simulink model "ex_codegen_dsp"  (R2013a)
settings: Solver=FixedStepDiscrete  SolverMode=SingleTasking  StartTime=0.0  StopTime=60  RelTol=1e-3
undefined symbols (not defined in the file or in its folder): fdesignblkfcn, gcbh, get
libraries: dspsrcs4 x2, dspadpt3 x1, dspsnks4 x1
CloseFcn:
  | clear filter_wts;
  | clear tout;
settings Model: Creator=The MathWorks Inc.  LastModifiedBy=mainster
settings DataIOCC: SignalLoggingSaveFormat=ModelDataLogs
settings OptimizationCC: ExpressionDepthLimit=2147483647
settings DebuggingCC: FcnCallInpInsideContextMsg=UseLocalSettings
settings RTWCC: GenerateReport=on  LaunchReport=on
settings GRTTargetCC: CombineOutputUpdateFcns=off  GRTInterface=on

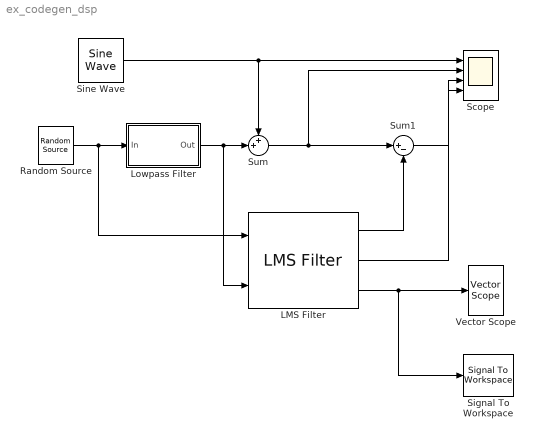
== system ex_codegen_dsp ==
  LMS Filter : dspadpt3/LMS Filter  Algo=Normalized LMS  L=32  stepflag=Dialog  mu=0.1  leakage=1.0  ic=0  Adapt=off  resetflag=None  weights=on  secondCoeffMode=User-defined  secondCoeffWordLength=2  secondCoeffFracLength=15  accum2Mode=User-defined  accum2FracLength=20  prodOutput2Mode=User-defined  prodOutput2FracLength=20  prodOutput3Mode=User-defined  prodOutput3FracLength=20  prodOutput4Mode=User-defined  prodOutput4FracLength=20  quotientMode=User-defined  quotientFracLength=20  roundingMode=Floor  overflowMode=off  addnparflag=off
  Lowpass Filter : Subsystem  DialogController=fdesignblkfcn  InitFcn=fdesignblkfcn(gcbh, {'InitFcn'});  mask(Lowpass Filter){}
      mask help: Design a lowpass filter
      settings: CopyFcn=fdesignblkfcn(gcbh, {'CopyFcn'});
      mask Help: helpview(mapfilelocation('dspblks'), 'dsplowpassfilter')
      mask Display: disp('Lowpass')
  Random Source : dspsrcs4/Random Source  SrcType=Gaussian  NormMethod=Ziggurat  CltLength=12  MinVal=0  MaxVal=1  MeanVal=0  VarVal=1  RepMode=Specify seed  rawSeed=[23341]  IsInherit=off  SampMode=Discrete  SampTime=0.05  SampFrame=1  DataType=Double  OutComplex=Real
  Scope : Scope  NumInputPorts=4
      settings: YMin=-5~-5~-5~-5  YMax=5~5~5~5  DataFormat=Structure
  Signal To Workspace : SignalToWorkspace  VariableName=filter_wts  Save2DMode=3-D array (concatenate along third dimension)
      settings: CopyFcn=dspblkcopystw(gcbh);
  Sine Wave : dspsrcs4/Sine Wave  Amplitude=1  Frequency=0.5  Phase=0  SampleMode=Discrete  OutComplex=Real  CompMethod=Trigonometric fcn  TableSize=Speed  SampleTime=0.05  SamplesPerFrame=1  ResetState=Restart at time zero  dataType=double  wordLen=16  udDataType=sfix(16)  fracBitsMode=Best precision  numFracBits=15  OutDataTypeStr=double  LastOutDataTypeStr=double
  Sum : Sum  Inputs=++|
  Sum1 : Sum  Inputs=|+-
  Vector Scope : dspsnks4/Vector Scope  ScopeProperties=on  Domain=Time  HorizSpan=1  DisplayProperties=off  AxisGrid=on  Memory=off  FrameNumber=on  AxisLegend=off  AxisZoom=on  OpenScopeAtSimStart=on  OpenScopeImmediately=off  FigPos=get(0,'defaultfigureposition')  AxisProperties=off  XUnits=Hertz  XRange=[0...Fs/2]  InheritXIncr=on  XIncr=1  XLabel=Time  XLimit=Auto  XMin=0  XMax=1  XStart=0  YUnits=dB  YLabel=Filter Weights  LineProperties=off  LineDisables=on  LineStyles=:  LineMarkers=.  LineColors=[0 0 1]  XAxisParamsVer=6.9
      settings: YMin=-0.2  YMax=0.6
  wires:
  Sine Wave/1 -> Scope/1, Sum/1
  Random Source/1 -> LMS Filter/1, Lowpass Filter/1(In)
  Sum/1 -> Scope/2, Sum1/1
  Lowpass Filter/1(Out) -> Sum/2, LMS Filter/2
  LMS Filter/1 -> Sum1/2
  Sum1/1 -> Scope/3
  LMS Filter/2 -> Scope/4
  LMS Filter/3 -> Vector Scope/1, Signal To Workspace/1

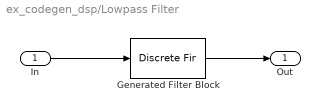
== system ex_codegen_dsp/Lowpass Filter ==
  In : Inport
  Generated Filter Block : DiscreteFir  Tag=BlockMethodSubSystem  Coefficients=[-0.00116169847246078432 -0.00138798082963417953 0.0019553437659341746 0.00292510641051443258 -0.00436604908256792157 -0.00635958912648804022 0.00900883950647731087 0.012454637566874099 -0.016904897878442366 -0.0226914396301924441 0.0303890031459586353 0.0410928751247308099 -0.0571719340677344853 -0.0848277531991029066 0.146887215886567446 0.449095734750016462 0.449095734750016462 0.146887215886567446 -0.0848277531991029066 -0.0571719340677344853 0.0410928751247308099 0.0303890031459586353 -0.0226914396301924441 -0.016904897878442366 0.012454637566874099 0.00900883950647731087 -0.00635958912648804022 -0.00436604908256792157 0.00292510641051443258 0.0019553437659341746 -0.00138798082963417953 -0.00116169847246078432]  InputProcessing=Columns as channels (frame based)
  Out : Outport
  wires:
  In/1 -> Generated Filter Block/1
  Generated Filter Block/1 -> Out/1
